simulink model "PM_block_control_FAST_syn_27_3"  (R2017a)
settings: Solver=ode4  StartTime=0.0  StopTime=100  FixedStep=0.0001  RelTol=1e-3
values from neighbouring files (symbols this model uses):
  Flux = 5.8264    [PM_1_5MW_syn_27.m]
  fs = 4000    [PM_1_5MW_syn_27.m]
  Id_set = 500    [PM_1_5MW_syn_27.m]
  Iq_set = 2200    [PM_1_5MW_syn_27.m]
  Ki = (Bandw/10*2*pi)*Kp    (= 0.0157079632679)    [PM_1_5MW_syn_27.m]
  Ki_Speed = Kp_Speed*2*pi*(BW/10)    (= 170820.076173)    [PM_1_5MW_syn_27.m]
  Kp = 1*.0005    (= 0.0005)    [PM_1_5MW_syn_27.m]
  Kp_Speed = 1.5*J/p*2*pi*BW    (= 5437.37190044)    [PM_1_5MW_syn_27.m]
  Ld = 0.001575    [PM_1_5MW_syn_27.m]
  Lq = 0.001575    [PM_1_5MW_syn_27.m]
  m = 1    [PM_1_5MW_syn_27.m]
  p = 26    [PM_1_5MW_syn_27.m]
  Rs = 0.000821    [PM_1_5MW_syn_27.m]
  Speed_set = w_m    (= 2.10172548525)    [PM_1_5MW_syn_27.m]
undefined symbols (not defined in the file or in its folder): Sollkurve_M_Optimum, Sollkurve_nGen_Optimum
libraries: powerlib x15, simulink x2
settings Model: Creator=Anjali  LastModifiedBy=sganzel
settings OptimizationCC: LifeSpan=inf
settings DebuggingCC: SFUnexpectedBacktrackingDiag=warning  SFNoUnconditionalDefaultTransitionDiag=warning  SFExecutionAtInitializationDiag=none
settings GRTTargetCC: TargetLangStandard=C89/C90 (ANSI)  GeneratePreprocessorConditionals=Disable all
settings ConfigComp: CovMetricSettings=dw  CovHtmlReporting=on  CovSaveCumulativeToWorkspaceVar=on  CovSaveSingleToWorkspaceVar=on  CovExternalEMLEnable=off

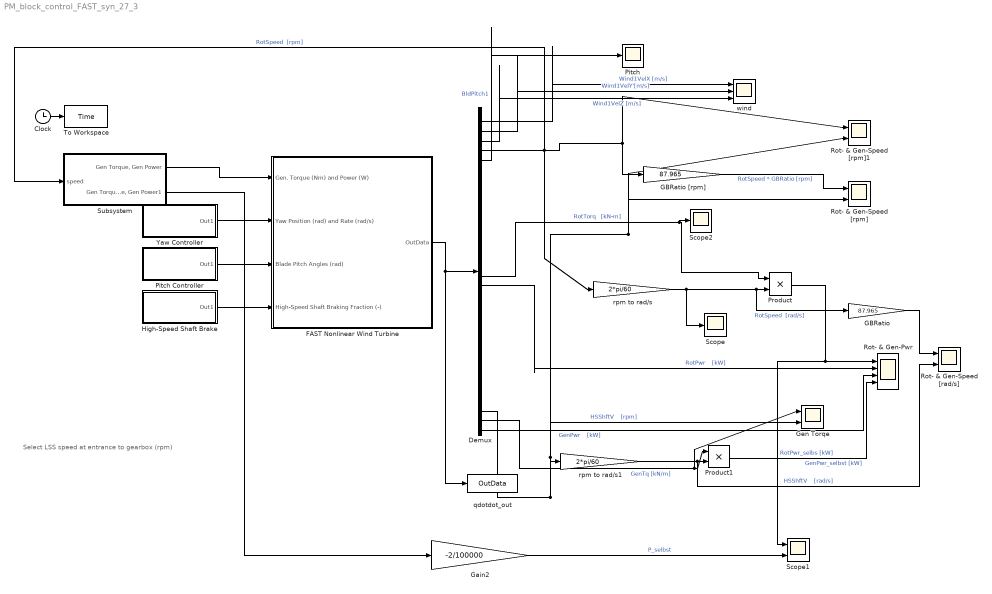
== system PM_block_control_FAST_syn_27_3 ==
  note: Select LSS speed at entrance to gearbox (rpm)
  Clock : Clock
  Demux : Demux  Outputs=34
  FAST Nonlinear Wind Turbine : Subsystem  mask(FAST Nonlinear Wind Turbine){}
      mask help: This block contains the FAST S-Function.
      mask init:
      | clear FAST_SFunc
  GBRatio : Gain  Gain=87.965
  GBRatio [rpm] : Gain  Gain=87.965
  Gain2 : Gain  Gain=-2/100000
  Gen Torqe : Scope  NumInputPorts=2
  High-Speed Shaft Brake : Subsystem
  Pitch : Scope
  Pitch Controller : Subsystem
  Product : Product
  Product1 : Product
  Rot- & Gen-Pwr : Scope  NumInputPorts=4
  Rot- & Gen-Speed [rad/s] : Scope  NumInputPorts=2
  Rot- & Gen-Speed [rpm] : Scope  NumInputPorts=2
  Rot- & Gen-Speed [rpm]1 : Scope  NumInputPorts=2
  Scope : Scope
  Scope1 : Scope  NumInputPorts=2
  Scope2 : Scope
  Subsystem : Subsystem
  To Workspace : ToWorkspace  VariableName=Time  SampleTime=-1
  Yaw Controller : Subsystem
  qdotdot_out : ToWorkspace  VariableName=OutData  SampleTime=-1
  rpm to rad/s : Gain  Gain=2*pi/60
  rpm to rad/s1 : Gain  Gain=2*pi/60
  wind : Scope  NumInputPorts=3
  wires:
  Clock/1 -> To Workspace/1
  Yaw Controller/1(Out1) -> FAST Nonlinear Wind Turbine/2(Yaw Position (rad) and Rate (rad/s))
  Pitch Controller/1(Out1) -> FAST Nonlinear Wind Turbine/3(Blade Pitch Angles (rad))
  FAST Nonlinear Wind Turbine/1(OutData) -> qdotdot_out/1, Demux/1
  High-Speed Shaft Brake/1(Out1) -> FAST Nonlinear Wind Turbine/4(High-Speed Shaft Braking Fraction (-))
  Demux/32 -> Gen Torqe/2, Rot- & Gen-Speed [rpm]1/2, Rot- & Gen-Speed [rpm]/2, rpm to rad/s1/1  "HSShftV    [rpm]"
  Demux/19 -> Rot- & Gen-Pwr/2  "RotPwr    [kW]"
  Demux/5 -> Rot- & Gen-Speed [rpm]1/1, GBRatio [rpm]/1, rpm to rad/s/1, Subsystem/1(speed)  "RotSpeed  [rpm]"
  Demux/18 -> Product/1, Scope2/1  "RotTorq   [kN-m]"
  Product/1 -> Scope1/1, Rot- & Gen-Pwr/1  "RotPwr_selbs [kW]"
  rpm to rad/s/1 -> Scope/1, GBRatio/1, Product/2  "RotSpeed  [rad/s]"
  Demux/34 -> Rot- & Gen-Pwr/3  "GenPwr    [kW]"
  Demux/33 -> Gen Torqe/1, Product1/1  "GenTq [kN/m]"
  rpm to rad/s1/1 -> Rot- & Gen-Speed [rad/s]/2, Product1/2  "HSShftV    [rad/s]"
  Product1/1 -> Rot- & Gen-Pwr/4  "GenPwr_selbst [kW]"
  GBRatio/1 -> Rot- & Gen-Speed [rad/s]/1
  GBRatio [rpm]/1 -> Rot- & Gen-Speed [rpm]/1  "RotSpeed * GBRatio [rpm]"
  Demux/2 -> wind/1  "Wind1VelX [m/s]"
  Demux/3 -> wind/2  "Wind1VelY [m/s]"
  Demux/4 -> wind/3  "Wind1VelZ [m/s]"
  Demux/6 -> Pitch/1  "BldPitch1"
  Subsystem/2("Gen Torque, Gen Power1") -> Gain2/1
  Gain2/1 -> Scope1/2  "P_selbst"
  Subsystem/1("Gen Torque, Gen Power") -> FAST Nonlinear Wind Turbine/1(Gen. Torque (Nm) and Power (W))

== system PM_block_control_FAST_syn_27_3/FAST Nonlinear Wind Turbine ==
  Gen. Torque (Nm) and Power (W) : Inport
  Yaw Position (rad) and Rate (rad/s) : Inport  Port=2
  Blade Pitch Angles (rad) : Inport  Port=3
  High-Speed Shaft Braking Fraction (-) : Inport  Port=4
  Mux1 : Mux
  S-Function : S-Function  FunctionName=FAST_SFunc  Parameters=FAST_InputFileName, TMax, 0  SFunctionDeploymentMode=off  EnableBusSupport=off
  Signal Specification1 : SignalSpecification  OutDataTypeStr=double  Dimensions=2
  Signal Specification2 : SignalSpecification  OutDataTypeStr=double  Dimensions=2
  OutData : Outport
  wires:
  Gen. Torque (Nm) and Power (W)/1 -> Signal Specification1/1
  S-Function/1 -> OutData/1
  Mux1/1 -> S-Function/1
  Blade Pitch Angles (rad)/1 -> Mux1/3
  Yaw Position (rad) and Rate (rad/s)/1 -> Signal Specification2/1
  Signal Specification1/1 -> Mux1/1
  Signal Specification2/1 -> Mux1/2
  High-Speed Shaft Braking Fraction (-)/1 -> Mux1/4

== system PM_block_control_FAST_syn_27_3/High-Speed Shaft Brake ==
  High-Speed Shaft Braking Fraction : Constant  Value=0
  Out1 : Outport
  wires:
  High-Speed Shaft Braking Fraction/1 -> Out1/1

== system PM_block_control_FAST_syn_27_3/Pitch Controller ==
  Blade Pitch Angles : Constant  Value=ones(1,3)'
  Pitch-winkel : Gain  Gain=0
  dergree2rad : Gain  Gain=2*pi/360
  Out1 : Outport
  wires:
  Blade Pitch Angles/1 -> Pitch-winkel/1
  Pitch-winkel/1 -> dergree2rad/1
  dergree2rad/1 -> Out1/1

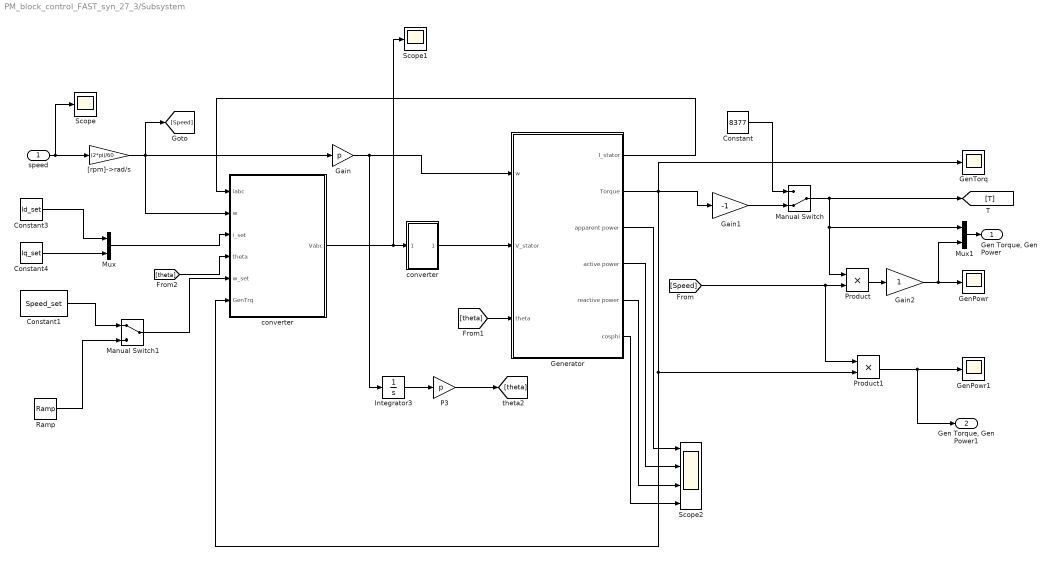
== system PM_block_control_FAST_syn_27_3/Subsystem ==
  speed : Inport
  Constant : Constant  Value=8377  VectorParams1D=off
  Constant1 : Constant  Value=Speed_set
  Constant3 : Constant  Value=Id_set
  Constant4 : Constant  Value=Iq_set
  Gain : Gain  Gain=p
  Gain1 : Gain  Gain=-1
  Gain2 : Gain
  GenPowr : Scope
  GenPowr1 : Scope
  GenTorq : Scope
  "Generator " : Subsystem
  Integrator3 : Integrator
  Manual Switch : ManualSwitch  CurrentSetting=0
  Manual Switch1 : ManualSwitch
  Mux : Mux  Inputs=2
  Mux1 : Mux  Inputs=2
  P3 : Gain  Gain=p
  Product : Product
  Product1 : Product
  Ramp : simulink/Sources/Ramp  slope=1/60*2*pi/10  start=40  X0=1.831548517042849
  Scope : Scope
  Scope1 : Scope
  Scope2 : Scope  NumInputPorts=4
  "[rpm]->rad/s" : Gain  Gain=(2*pi)/60
  converter : Subsystem
  "converter " : Subsystem
  "Gen Torque, Gen Power" : Outport
  "Gen Torque, Gen Power1" : Outport  Port=2
  wires:
  speed/1 -> Scope/1, "[rpm]->rad/s"/1
  "Generator "/1("I_stator ") -> "converter "/1(iabc)
  Constant3/1 -> Mux/1
  "Generator "/5(reactive power) -> Scope2/3
  [theta] -> "converter "/4(theta)
  Constant4/1 -> Mux/2
  "Generator "/6(cosphi) -> Scope2/4
  "Generator "/3(apparent power) -> Scope2/1
  "converter "/1(Vabc) -> Scope1/1, converter/1(iabc)
  "Generator "/4(active power) -> Scope2/2
  Constant1/1 -> Manual Switch1/1
  [theta] -> "Generator "/3("theta ")
  Mux/1 -> "converter "/3(i_set)
  Gain/1 -> Integrator3/1, "Generator "/1(w)
  "[rpm]->rad/s"/1 -> [Speed], Gain/1, "converter "/2(w)
  Integrator3/1 -> P3/1
  P3/1 -> [theta]
  [Speed] -> Product/2, Product1/1
  Product1/1 -> "Gen Torque, Gen Power1"/1, GenPowr1/1
  Mux1/1 -> "Gen Torque, Gen Power"/1
  Product/1 -> Gain2/1
  Constant/1 -> Manual Switch/1
  Gain2/1 -> GenPowr/1, Mux1/2
  "Generator "/2(Torque) -> Gain1/1, "converter "/6(GenTrq), Product1/2, GenTorq/1
  Manual Switch/1 -> [T], Mux1/1, Product/1
  Manual Switch1/1 -> "converter "/5(w_set)
  Ramp/1 -> Manual Switch1/2
  Gain1/1 -> Manual Switch/2
  converter/1(v_abc) -> "Generator "/2("V_stator ")

== system PM_block_control_FAST_syn_27_3/Yaw Controller ==
  Mux : Mux  Inputs=2
  Yaw Position : Constant  Value=0
  Yaw rate : Constant  Value=0
  Out1 : Outport
  wires:
  Mux/1 -> Out1/1
  Yaw Position/1 -> Mux/1
  Yaw rate/1 -> Mux/2

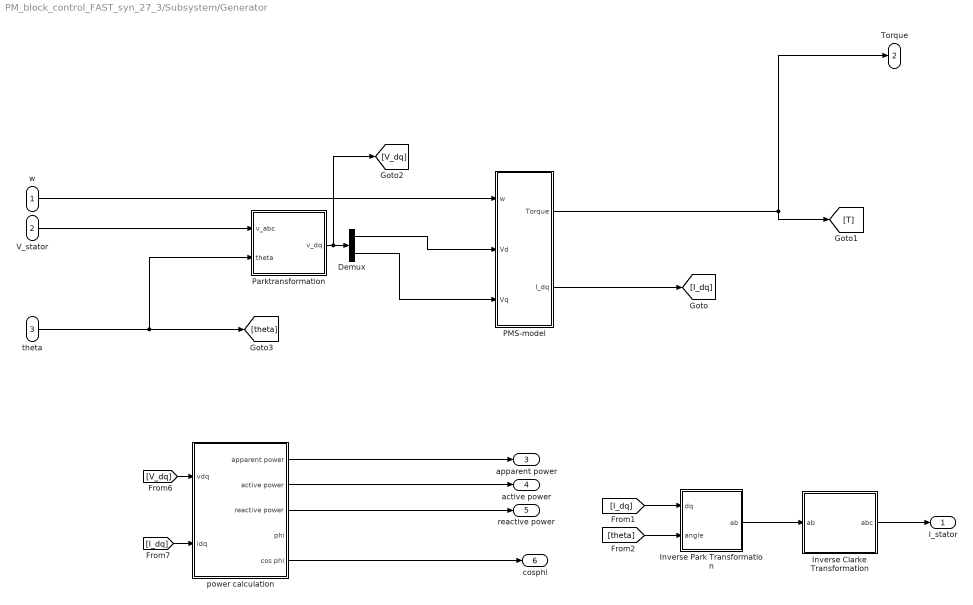
== system PM_block_control_FAST_syn_27_3/Subsystem/Generator  ==
  w : Inport
  "V_stator " : Inport  Port=2
  "theta " : Inport  Port=3
  Demux : Demux  Outputs=2
  Inverse Clarke Transformation : Subsystem
  Inverse Park Transformation : Subsystem
  PMS-model : Subsystem
  Parktransformation : Subsystem
  power calculation : Subsystem
  "I_stator " : Outport
  Torque : Outport  Port=2
  apparent power : Outport  Port=3
  active power : Outport  Port=4
  reactive power : Outport  Port=5
  cosphi : Outport  Port=6
  wires:
  PMS-model/2(I_dq) -> [I_dq]
  PMS-model/1(Torque) -> [T], Torque/1
  "V_stator "/1 -> Parktransformation/1(v_abc)
  "theta "/1 -> [theta], Parktransformation/2(theta)
  Parktransformation/1(v_dq) -> [V_dq], Demux/1
  Demux/1 -> PMS-model/2(Vd)
  Demux/2 -> PMS-model/3(Vq)
  w/1 -> PMS-model/1(w)
  Inverse Park Transformation/1(ab) -> Inverse Clarke Transformation/1(ab)
  [I_dq] -> Inverse Park Transformation/1(dq)
  Inverse Clarke Transformation/1(abc) -> "I_stator "/1
  [theta] -> Inverse Park Transformation/2(angle)
  [V_dq] -> power calculation/1(vdq)
  [I_dq] -> power calculation/2(idq)
  power calculation/3(reactive power) -> reactive power/1
  power calculation/2(active power) -> active power/1
  power calculation/1(apparent power) -> apparent power/1
  power calculation/5(cos phi) -> cosphi/1

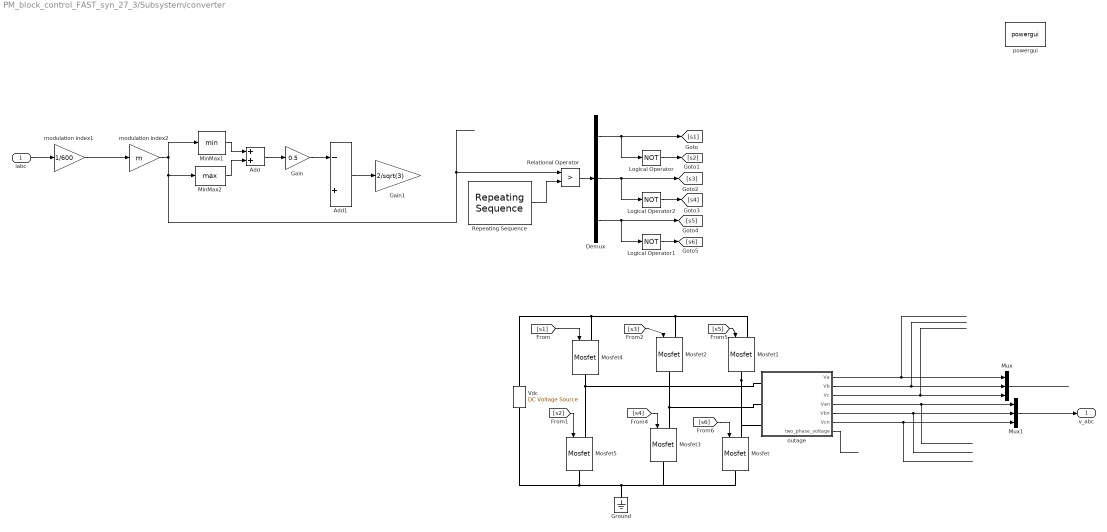
== system PM_block_control_FAST_syn_27_3/Subsystem/converter ==
  iabc : Inport
  Add : Sum
  Add1 : Sum  Inputs=-+
  Demux : Demux  Outputs=3
  Gain : Gain  Gain=0.5
  Gain1 : Gain  Gain=2/sqrt(3)
  Ground : powerlib/Elements/Ground  LConnTagsString=a
  Logical Operator : Logic  Operator=NOT  AllPortsSameDT=off  OutDataTypeStr=boolean
  Logical Operator1 : Logic  Operator=NOT  AllPortsSameDT=off  OutDataTypeStr=boolean
  Logical Operator2 : Logic  Operator=NOT  AllPortsSameDT=off  OutDataTypeStr=boolean
  MinMax1 : MinMax  SaturateOnIntegerOverflow=on  InputSameDT=on
  MinMax2 : MinMax  Function=max  SaturateOnIntegerOverflow=on  InputSameDT=on
  Mosfet{,1..5} (6 alike) : powerlib/Power Electronics/Mosfet  Ron=0.1  Lon=0  Rd=0.01  Vfd=0  IC=0  Rs=1e5  Cs=inf  Measurements=off
  Mux : Mux  Inputs=3
  Mux1 : Mux  Inputs=3
  Relational Operator : RelationalOperator  Operator=>  RndMeth=Nearest
  Repeating Sequence : simulink/Sources/Repeating Sequence  rep_seq_t=[0 0.25/fs 0.5/fs 0.75/fs 1/fs]  rep_seq_y=[1 0 -1 0 1]
  Vdc : powerlib/Electrical Sources/DC Voltage Source  Amplitude=1200  Measurements=None
  modulation index1 : Gain  Gain=1/600  SaturateOnIntegerOverflow=on  OutDataTypeStr=Inherit: Same as input  ParamDataTypeStr=Inherit: Same as input
  modulation index2 : Gain  Gain=m  SaturateOnIntegerOverflow=on  OutDataTypeStr=Inherit: Same as input  ParamDataTypeStr=Inherit: Same as input
  outage : Subsystem
  powergui : powerlib/powergui  Priority=1  SimulationMode=Continuous  SampleTime=50e-6  frequency=60  Iterations=50  frequencyindice=0  Pbase=100e6  ErrMax=1e-4  UnitsV=kV  UnitsW=MW  buscounter=0  FunctionMessages=off  echomessages=off  EnableUseOfTLC=off  CurrentSourceSwitches=on  DisableSnubberDevices=off  DisableRonSwitches=off  DisableVfSwitches=off  DisplayEquations=off  SolverType=Tustin/Backward Euler (TBE)  Interpol=off  ExternalGateDelay=off  methode=off  Ts=100  x0status=blocks  SPID=off  SwTol=0  HookPort=off  RestoreLinks=warning  ResistiveCurrentMeasurement=off  Frange=[0:2:500]  Ylog=off  Xlog=on  ShowGrid=off  save=off  variable=ZData  structure=Filtered_voltages  ZoomFFT=off  StartTime=0.02  cycles=1  DisplayStyle=1  fundamental=50  FreqAxis=off  MaxFrequency=1000  frequencyindicesteady=1  RmsSteady=1  display=off
  v_abc : Outport
  wires:
  Mux/1 -> ?
  Add1/1 -> Gain1/1
  Gain/1 -> Add1/1
  MinMax2/1 -> Add/2
  Add/1 -> Gain/1
  iabc/1 -> modulation index1/1
  MinMax1/1 -> Add/1
  Demux/2 -> [s3], Logical Operator2/1
  Demux/3 -> [s5], Logical Operator1/1
  Logical Operator1/1 -> [s6]
  Logical Operator/1 -> [s2]
  Logical Operator2/1 -> [s4]
  Demux/1 -> [s1], Logical Operator/1
  modulation index2/1 -> MinMax1/1, Relational Operator/1, MinMax2/1
  Relational Operator/1 -> Demux/1
  Repeating Sequence/1 -> Relational Operator/2
  outage/2(Vb) -> Mux/2
  [s3] -> Mosfet2/1
  outage/1(Va) -> Mux/1
  [s6] -> Mosfet/1
  [s2] -> Mosfet5/1
  [s5] -> Mosfet1/1
  [s4] -> Mosfet3/1
  [s1] -> Mosfet4/1
  outage/3(Vc) -> Mux/3
  outage/7(two_phase_voltage) -> ?
  modulation index1/1 -> modulation index2/1
  outage/6(Vcn) -> Mux1/3
  Mux1/1 -> v_abc/1
  outage/5(Vbn) -> Mux1/2
  outage/4(Van) -> Mux1/1
  connections:
  Mosfet5/RConn1 -- Vdc/LConn1 -- Ground/LConn1 -- Mosfet/RConn1 -- Mosfet3/RConn1
  Mosfet1/LConn1 -- Vdc/RConn1 -- Mosfet4/LConn1 -- Mosfet2/LConn1
  Mosfet5/LConn1 -- outage/LConn1 -- Mosfet4/RConn1
  Mosfet2/RConn1 -- Mosfet3/LConn1 -- outage/LConn2
  Mosfet1/RConn1 -- outage/LConn3 -- Mosfet/LConn1

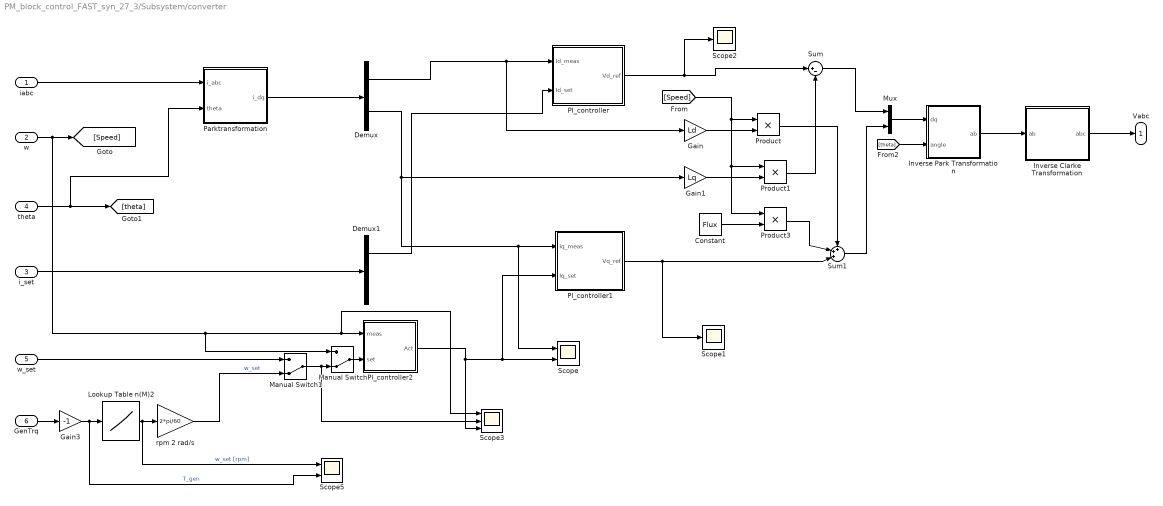
== system PM_block_control_FAST_syn_27_3/Subsystem/converter  ==
  iabc : Inport
  w : Inport  Port=2
  i_set : Inport  Port=3
  theta : Inport  Port=4
  w_set : Inport  Port=5
  GenTrq : Inport  Port=6
  Constant : Constant  Value=Flux
  Demux : Demux  Outputs=2
  Demux1 : Demux  Outputs=2
  Gain : Gain  Gain=Ld
  Gain1 : Gain  Gain=Lq
  Gain3 : Gain  Gain=-1
  Inverse Clarke Transformation : Subsystem
  Inverse Park Transformation : Subsystem
  Lookup Table n(M)2 : Lookup_n-D  NumberOfTableDimensions=1  BreakpointsForDimension1=Sollkurve_M_Optimum  Table=Sollkurve_nGen_Optimum  InternalRulePriority=Speed  RndMeth=Simplest  InputSameDT=on
  Manual Switch : ManualSwitch  CurrentSetting=0
  Manual Switch1 : ManualSwitch  CurrentSetting=0
  Mux : Mux  Inputs=2
  PI_controller : Subsystem
  PI_controller1 : Subsystem
  PI_controller2 : Subsystem
  Parktransformation : Subsystem
  Product : Product
  Product1 : Product
  Product3 : Product
  Scope : Scope  NumInputPorts=2
  Scope1 : Scope
  Scope2 : Scope
  Scope3 : Scope  NumInputPorts=3
  Scope5 : Scope  NumInputPorts=2
  Sum : Sum  Inputs=|+-
  Sum1 : Sum  Inputs=+++|
  rpm 2 rad/s : Gain  Gain=2*pi/60
  Vabc : Outport
  wires:
  iabc/1 -> Parktransformation/1(i_abc)
  Parktransformation/1(i_dq) -> Demux/1
  Demux/1 -> Gain/1, PI_controller/1(Id_meas)
  Demux/2 -> Gain1/1, Scope/1, PI_controller1/1(Iq_meas)
  i_set/1 -> Demux1/1
  Demux1/1 -> PI_controller/2(Id_set)
  Gain/1 -> Product/2
  Gain1/1 -> Product1/2
  [Speed] -> Product/1, Product3/1, Product1/1
  PI_controller/1(Vd_ref) -> Scope2/1, Sum/1
  Product1/1 -> Sum/2
  Product/1 -> Sum1/1
  Inverse Park Transformation/1(ab) -> Inverse Clarke Transformation/1(ab)
  Inverse Clarke Transformation/1(abc) -> Vabc/1
  Sum/1 -> Mux/1
  Sum1/1 -> Mux/2
  Mux/1 -> Inverse Park Transformation/1(dq)
  theta/1 -> Parktransformation/2(theta), [theta]
  [theta] -> Inverse Park Transformation/2(angle)
  PI_controller1/1(Vq_ref) -> Scope1/1, Sum1/3
  Constant/1 -> Product3/2
  Product3/1 -> Sum1/2
  w/1 -> Scope3/1, PI_controller2/1(meas), Manual Switch/1, [Speed]
  Manual Switch/1 -> PI_controller2/2(set)
  PI_controller2/1(Act) -> Scope/2, PI_controller1/2(Iq_set), Scope3/3
  Gain3/1 -> Scope5/2, Lookup Table n(M)2/1  "T_gen"
  rpm 2 rad/s/1 -> Manual Switch1/2  "w_set"
  w_set/1 -> Manual Switch1/1
  Manual Switch1/1 -> Scope3/2, Manual Switch/2
  Lookup Table n(M)2/1 -> Scope5/1, rpm 2 rad/s/1  "w_set [rpm]"
  GenTrq/1 -> Gain3/1

== system PM_block_control_FAST_syn_27_3/Subsystem/Generator /Inverse Clarke Transformation ==
  ab : Inport
  Demux : Demux  Outputs=2
  Gain1 : Gain  Gain=1/2
  Gain2 : Gain  Gain=sqrt(3)
  Gain4 : Gain  Gain=1/2
  Mux : Mux  Inputs=3
  Sum : Sum  Inputs=|-+
  Sum1 : Sum  Inputs=|--
  abc : Outport
  wires:
  Mux/1 -> abc/1
  ab/1 -> Demux/1
  Sum1/1 -> Gain1/1
  Sum/1 -> Gain4/1
  Gain2/1 -> Sum1/2, Sum/2
  Demux/1 -> Sum1/1, Sum/1, Mux/1
  Demux/2 -> Gain2/1
  Gain4/1 -> Mux/2
  Gain1/1 -> Mux/3

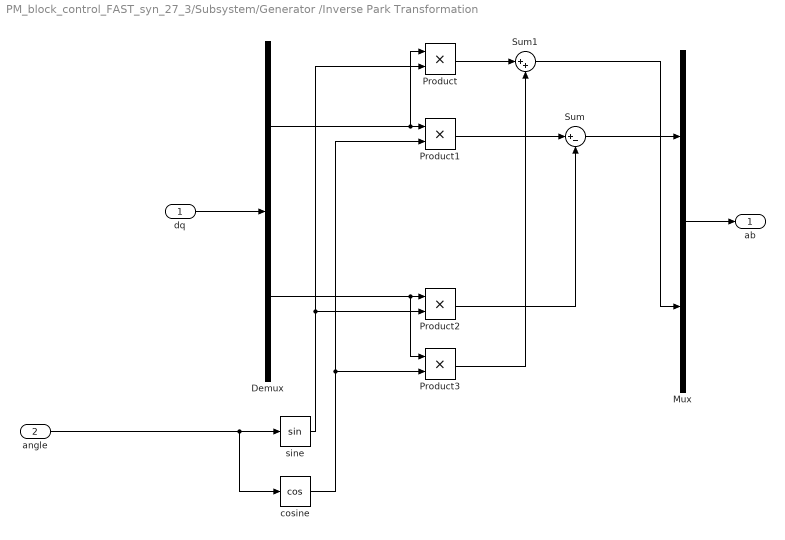
== system PM_block_control_FAST_syn_27_3/Subsystem/Generator /Inverse Park Transformation ==
  dq : Inport
  angle : Inport  Port=2
  Demux : Demux  Outputs=2
  Mux : Mux  Inputs=2
  Product{,1..3} (4 alike) : Product  RndMeth=Zero
  Sum : Sum  Inputs=|+-
  Sum1 : Sum  Inputs=|++
  cosine : Trigonometry  Operator=cos
  sine : Trigonometry
  ab : Outport
  wires:
  Sum1/1 -> Mux/2
  Sum/1 -> Mux/1
  Product2/1 -> Sum/2
  Product1/1 -> Sum/1
  Product3/1 -> Sum1/2
  Product/1 -> Sum1/1
  cosine/1 -> Product3/2, Product1/2
  sine/1 -> Product2/2, Product/2
  Demux/2 -> Product3/1, Product2/1
  Demux/1 -> Product1/1, Product/1
  Mux/1 -> ab/1
  dq/1 -> Demux/1
  angle/1 -> cosine/1, sine/1

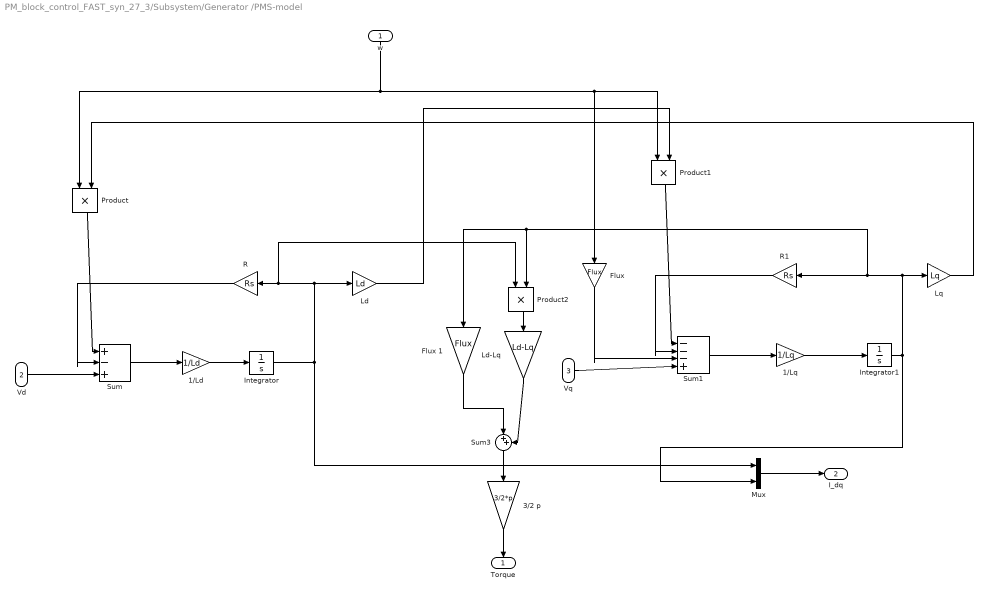
== system PM_block_control_FAST_syn_27_3/Subsystem/Generator /PMS-model ==
  w : Inport
  Vd : Inport  Port=2
  Vq : Inport  Port=3
  1/Ld : Gain  Gain=1/Ld
  1/Lq : Gain  Gain=1/Lq
  3/2 p : Gain  Gain=3/2*p
  "Flux " : Gain  Gain=Flux
  Flux 1 : Gain  Gain=Flux
  Integrator : Integrator
  Integrator1 : Integrator
  Ld : Gain  Gain=Ld
  Ld-Lq : Gain  Gain=Ld-Lq
  Lq : Gain  Gain=Lq
  Mux : Mux  Inputs=2
  Product : Product
  Product1 : Product
  Product2 : Product
  R : Gain  Gain=Rs
  R1 : Gain  Gain=Rs
  Sum : Sum  Inputs=|+-+
  Sum1 : Sum  Inputs=|---+
  Sum3 : Sum  Inputs=|++
  Torque : Outport
  I_dq : Outport  Port=2
  wires:
  R/1 -> Sum/2
  Product1/1 -> Sum1/1
  w/1 -> "Flux "/1, Product1/1, Product/1
  Vd/1 -> Sum/3
  3/2 p/1 -> Torque/1
  Mux/1 -> I_dq/1
  Product/1 -> Sum/1
  Sum3/1 -> 3/2 p/1
  R1/1 -> Sum1/2
  Sum/1 -> 1/Ld/1
  1/Ld/1 -> Integrator/1
  Integrator/1 -> Product2/1, R/1, Ld/1, Mux/1
  Sum1/1 -> 1/Lq/1
  1/Lq/1 -> Integrator1/1
  Integrator1/1 -> Product2/2, Flux 1/1, R1/1, Lq/1, Mux/2
  Ld/1 -> Product1/2
  Lq/1 -> Product/2
  Vq/1 -> Sum1/4
  "Flux "/1 -> Sum1/3
  Flux 1/1 -> Sum3/1
  Ld-Lq/1 -> Sum3/2
  Product2/1 -> Ld-Lq/1

== system PM_block_control_FAST_syn_27_3/Subsystem/Generator /Parktransformation ==
  v_abc : Inport
  theta : Inport  Port=2
  Scope1 : Scope
  Scope2 : Scope
  Scope3 : Scope
  Three-phase current : Subsystem
  abc to alpha-beta : Subsystem
  alpha-beta to dq : Subsystem
  f : Constant  Value=50
  f1 : Constant  Value=20
  v_dq : Outport
  wires:
  abc to alpha-beta/1("alpha-beta ") -> Scope1/1, alpha-beta to dq/2("alpha-beta ")
  alpha-beta to dq/1(Out1) -> v_dq/1, Scope2/1
  f1/1 -> Three-phase current/2(In2)
  v_abc/1 -> Scope3/1, abc to alpha-beta/1(abc)
  theta/1 -> alpha-beta to dq/1(theta)

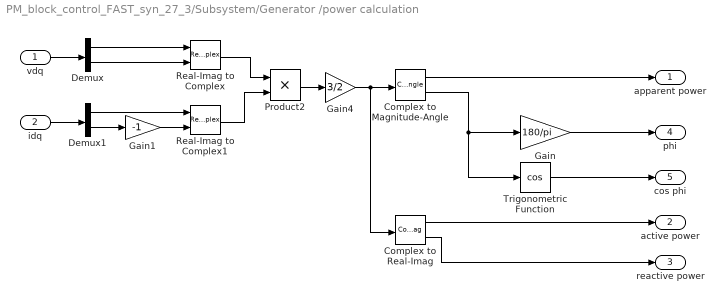
== system PM_block_control_FAST_syn_27_3/Subsystem/Generator /power calculation ==
  vdq : Inport
  idq : Inport  Port=2
  Complex to Magnitude-Angle : ComplexToMagnitudeAngle
  Complex to Real-Imag : ComplexToRealImag
  Demux : Demux  Outputs=2
  Demux1 : Demux  Outputs=2
  Gain : Gain  Gain=180/pi
  Gain1 : Gain  Gain=-1
  Gain4 : Gain  Gain=3/2
  Product2 : Product  RndMeth=Zero
  Real-Imag to Complex : RealImagToComplex
  Real-Imag to Complex1 : RealImagToComplex
  Trigonometric Function : Trigonometry  Operator=cos
  apparent power : Outport
  active power : Outport  Port=2
  reactive power : Outport  Port=3
  phi : Outport  Port=4
  cos phi : Outport  Port=5
  wires:
  Demux/1 -> Real-Imag to Complex/1
  Demux/2 -> Real-Imag to Complex/2
  Demux1/1 -> Real-Imag to Complex1/1
  Real-Imag to Complex/1 -> Product2/1
  Real-Imag to Complex1/1 -> Product2/2
  Product2/1 -> Gain4/1
  vdq/1 -> Demux/1
  idq/1 -> Demux1/1
  Complex to Magnitude-Angle/1 -> apparent power/1
  Complex to Magnitude-Angle/2 -> Trigonometric Function/1, Gain/1
  Gain/1 -> phi/1
  Demux1/2 -> Gain1/1
  Gain1/1 -> Real-Imag to Complex1/2
  Trigonometric Function/1 -> cos phi/1
  Complex to Real-Imag/1 -> active power/1
  Complex to Real-Imag/2 -> reactive power/1
  Gain4/1 -> Complex to Real-Imag/1, Complex to Magnitude-Angle/1

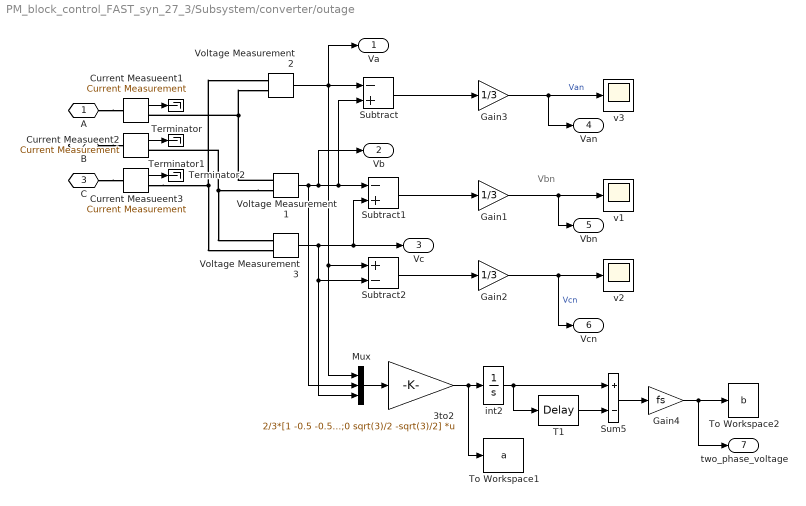
== system PM_block_control_FAST_syn_27_3/Subsystem/converter/outage ==
  note: Vbn
  3to2 : Gain  Gain=2/3*[1 -0.5 -0.5;0 sqrt(3)/2 -sqrt(3)/2]  Multiplication=Matrix(K*u)  SaturateOnIntegerOverflow=on  OutDataTypeStr=Inherit: Same as input  ParamDataTypeStr=Inherit: Same as input
  Current Measueent1 : powerlib/Measurements/Current Measurement  PhasorSimulation=off  OutputType=Complex  PSBequivalent=0
  Current Measueent2 : powerlib/Measurements/Current Measurement  PhasorSimulation=off  OutputType=Complex  PSBequivalent=0
  Current Measueent3 : powerlib/Measurements/Current Measurement  PhasorSimulation=off  OutputType=Complex  PSBequivalent=0
  Gain1 : Gain  Gain=1/3
  Gain2 : Gain  Gain=1/3
  Gain3 : Gain  Gain=1/3
  Gain4 : Gain  Gain=fs  SaturateOnIntegerOverflow=on  OutDataTypeStr=Inherit: Same as input  ParamDataTypeStr=Inherit: Same as input
  Mux : Mux  Inputs=3
  Subtract : Sum  Inputs=-+
  Subtract1 : Sum  Inputs=-+
  Subtract2 : Sum  Inputs=+-
  Sum5 : Sum  Inputs=+-  SaturateOnIntegerOverflow=on  InputSameDT=on  OutDataTypeStr=Inherit: Same as first input
  T1 : TransportDelay  DelayTime=1/fs  BufferSize=2048
  Terminator : Terminator
  Terminator1 : Terminator
  Terminator2 : Terminator
  To Workspace1 : ToWorkspace  VariableName=a  SampleTime=-1
      settings: Decimation=2
  To Workspace2 : ToWorkspace  VariableName=b  SampleTime=-1
      settings: Decimation=2
  Voltage Measurement1 : powerlib/Measurements/Voltage Measurement  PhasorSimulation=off  OutputType=Complex  PSBequivalent=0
  Voltage Measurement2 : powerlib/Measurements/Voltage Measurement  PhasorSimulation=off  OutputType=Complex  PSBequivalent=0
  Voltage Measurement3 : powerlib/Measurements/Voltage Measurement  PhasorSimulation=off  OutputType=Complex  PSBequivalent=0
  int2 : Integrator
  v1 : Scope
  v2 : Scope
  v3 : Scope
  A : PMIOPort  Port=1  Side=Left
  B : PMIOPort  Port=2  Side=Left
  C : PMIOPort  Port=3  Side=Left
  Va : Outport
  Vb : Outport  Port=2
  Vc : Outport  Port=3
  Van : Outport  Port=4
  Vbn : Outport  Port=5
  Vcn : Outport  Port=6
  two_phase_voltage : Outport  Port=7
  wires:
  Gain2/1 -> v2/1, Vcn/1  "Vcn"
  Subtract2/1 -> Gain2/1
  Gain1/1 -> v1/1, Vbn/1
  Subtract1/1 -> Gain1/1
  Voltage Measurement3/1 -> Subtract1/2, Vc/1, Subtract2/2, Mux/3
  Gain3/1 -> v3/1, Van/1  "Van"
  Subtract/1 -> Gain3/1
  Voltage Measurement1/1 -> Subtract/2, Subtract1/1, Vb/1, Mux/2
  Voltage Measurement2/1 -> Subtract/1, Va/1, Subtract2/1, Mux/1
  Current Measueent1/1 -> Terminator/1
  Current Measueent2/1 -> Terminator1/1
  Current Measueent3/1 -> Terminator2/1
  Mux/1 -> 3to2/1
  3to2/1 -> int2/1, To Workspace1/1
  T1/1 -> Sum5/2
  int2/1 -> Sum5/1, T1/1
  Sum5/1 -> Gain4/1
  Gain4/1 -> To Workspace2/1, two_phase_voltage/1
  connections:
  Voltage Measurement1/LConn1 -- Current Measueent1/RConn1 -- Voltage Measurement2/LConn2
  Voltage Measurement1/LConn2 -- Current Measueent2/RConn1 -- Voltage Measurement3/LConn1
  Current Measueent3/RConn1 -- Voltage Measurement2/LConn1 -- Voltage Measurement3/LConn2
  A/RConn1 -- Current Measueent1/LConn1
  B/RConn1 -- Current Measueent2/LConn1
  C/RConn1 -- Current Measueent3/LConn1

== system PM_block_control_FAST_syn_27_3/Subsystem/converter /Inverse Clarke Transformation ==
  ab : Inport
  Demux : Demux  Outputs=2
  Gain1 : Gain  Gain=1/2
  Gain2 : Gain  Gain=sqrt(3)
  Gain4 : Gain  Gain=1/2
  Mux : Mux  Inputs=3
  Sum : Sum  Inputs=|-+
  Sum1 : Sum  Inputs=|--
  abc : Outport
  wires:
  Mux/1 -> abc/1
  ab/1 -> Demux/1
  Sum1/1 -> Gain1/1
  Sum/1 -> Gain4/1
  Gain2/1 -> Sum1/2, Sum/2
  Demux/1 -> Sum1/1, Sum/1, Mux/1
  Demux/2 -> Gain2/1
  Gain4/1 -> Mux/2
  Gain1/1 -> Mux/3

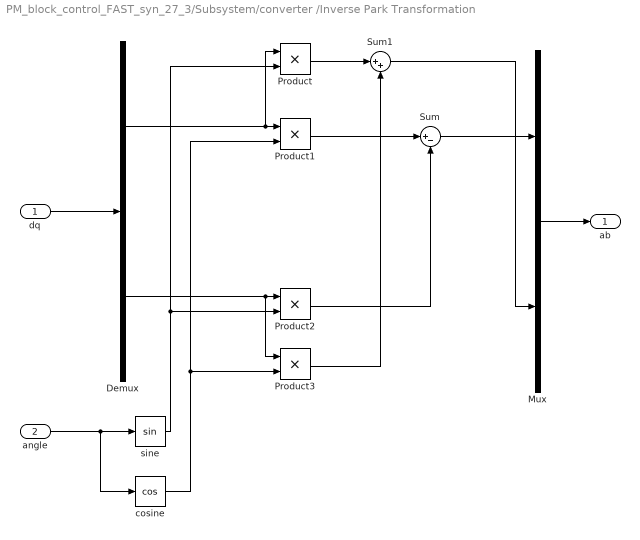
== system PM_block_control_FAST_syn_27_3/Subsystem/converter /Inverse Park Transformation ==
  dq : Inport
  angle : Inport  Port=2
  Demux : Demux  Outputs=2
  Mux : Mux  Inputs=2
  Product{,1..3} (4 alike) : Product  RndMeth=Zero
  Sum : Sum  Inputs=|+-
  Sum1 : Sum  Inputs=|++
  cosine : Trigonometry  Operator=cos
  sine : Trigonometry
  ab : Outport
  wires:
  Sum1/1 -> Mux/2
  Sum/1 -> Mux/1
  Product2/1 -> Sum/2
  Product1/1 -> Sum/1
  Product3/1 -> Sum1/2
  Product/1 -> Sum1/1
  angle/1 -> cosine/1, sine/1
  cosine/1 -> Product3/2, Product1/2
  sine/1 -> Product2/2, Product/2
  Demux/2 -> Product3/1, Product2/1
  Demux/1 -> Product1/1, Product/1
  Mux/1 -> ab/1
  dq/1 -> Demux/1

== system PM_block_control_FAST_syn_27_3/Subsystem/converter /PI_controller ==
  Id_meas : Inport
  Id_set : Inport  Port=2
  Gain : Gain  Gain=Kp
  Gain1 : Gain  Gain=Ki
  Integrator : Integrator
  Sum : Sum  Inputs=|++
  Sum1 : Sum  Inputs=|-+
  "id " : Scope  NumInputPorts=2
  Vd_ref : Outport
  wires:
  Gain/1 -> Sum/1
  Integrator/1 -> Sum/2
  Sum1/1 -> Gain1/1, Gain/1
  Id_meas/1 -> "id "/1, Sum1/1
  Id_set/1 -> "id "/2, Sum1/2
  Sum/1 -> Vd_ref/1
  Gain1/1 -> Integrator/1

== system PM_block_control_FAST_syn_27_3/Subsystem/converter /PI_controller1 ==
  Iq_meas : Inport
  Iq_set : Inport  Port=2
  Gain : Gain  Gain=Kp
  Gain1 : Gain  Gain=Ki
  Integrator : Integrator
  Sum : Sum  Inputs=|++
  Sum1 : Sum  Inputs=|-+
  iq : Scope  NumInputPorts=2
  Vq_ref : Outport
  wires:
  Gain1/1 -> Integrator/1
  Sum/1 -> Vq_ref/1
  Iq_set/1 -> iq/1, Sum1/2
  Sum1/1 -> Gain/1, Gain1/1
  Integrator/1 -> Sum/2
  Gain/1 -> Sum/1
  Iq_meas/1 -> iq/2, Sum1/1

== system PM_block_control_FAST_syn_27_3/Subsystem/converter /PI_controller2 ==
  meas : Inport
  set : Inport  Port=2
  Gain : Gain  Gain=Kp_Speed
  Gain1 : Gain  Gain=Ki_Speed
  Integrator : Integrator
  Sum : Sum  Inputs=|++
  Sum1 : Sum  Inputs=|-+
  "speed " : Scope  NumInputPorts=2
  Act : Outport
  wires:
  Gain1/1 -> Integrator/1
  Sum/1 -> Act/1
  Sum1/1 -> Gain1/1, Gain/1
  Integrator/1 -> Sum/2
  Gain/1 -> Sum/1
  set/1 -> "speed "/1, Sum1/2
  meas/1 -> "speed "/2, Sum1/1

== system PM_block_control_FAST_syn_27_3/Subsystem/converter /Parktransformation ==
  i_abc : Inport
  theta : Inport  Port=2
  3phase to ab : Subsystem
  alpha-beta to dq : Subsystem
  i_dq : Outport
  wires:
  3phase to ab/1(Out1) -> alpha-beta to dq/2("alpha-beta ")
  alpha-beta to dq/1(Out1) -> i_dq/1
  i_abc/1 -> 3phase to ab/1(In1)
  theta/1 -> alpha-beta to dq/1(theta)

== system PM_block_control_FAST_syn_27_3/Subsystem/Generator /Parktransformation/Three-phase current ==
  In1 : Inport
  In2 : Inport  Port=2
  Constant3 : Constant  Value=2*pi/3
  Constant4 : Constant  Value=-2*pi/3
  Gain : Gain  Gain=2*pi
  Integrator : Integrator
  Mux : Mux  Inputs=3
  Product : Product
  Sum : Sum  Inputs=|++
  Sum1 : Sum  Inputs=|++
  Trigonometric Function : Trigonometry  Operator=cos
  "abc " : Outport
  wires:
  Constant4/1 -> Sum1/2
  Trigonometric Function/1 -> Product/1
  Gain/1 -> Integrator/1
  In1/1 -> Gain/1
  In2/1 -> Product/2
  Sum/1 -> Mux/2
  Constant3/1 -> Sum/2
  Sum1/1 -> Mux/3
  Mux/1 -> Trigonometric Function/1
  Integrator/1 -> Sum/1, Sum1/1, Mux/1
  Product/1 -> "abc "/1

== system PM_block_control_FAST_syn_27_3/Subsystem/Generator /Parktransformation/abc to alpha-beta ==
  abc : Inport
  Demux : Demux  Outputs=3
  Gain : Gain  Gain=1/sqrt(3)
  Mux : Mux  Inputs=2
  Sum : Sum  Inputs=|+-
  "alpha-beta " : Outport
  wires:
  abc/1 -> Demux/1
  Sum/1 -> Gain/1
  Demux/2 -> Sum/1
  Demux/3 -> Sum/2
  Gain/1 -> Mux/2
  Demux/1 -> Mux/1
  Mux/1 -> "alpha-beta "/1

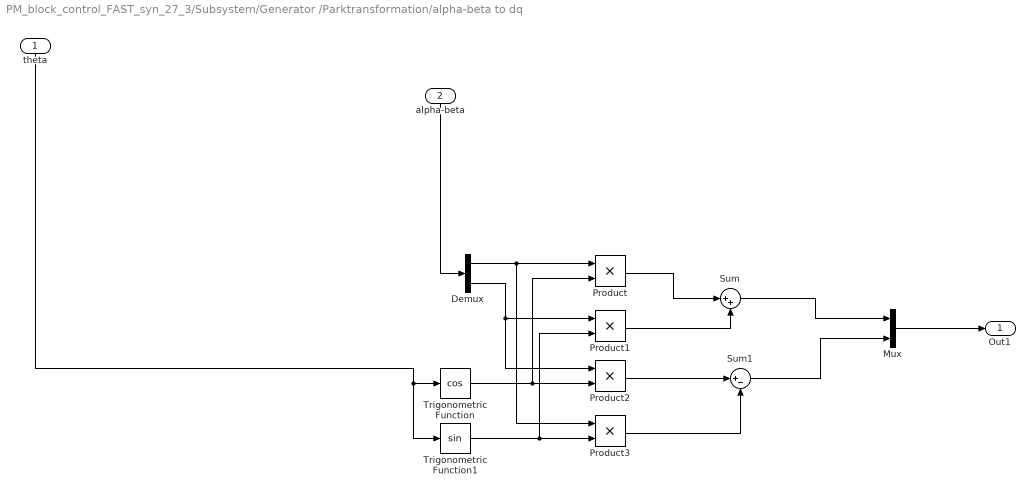
== system PM_block_control_FAST_syn_27_3/Subsystem/Generator /Parktransformation/alpha-beta to dq ==
  theta : Inport
  "alpha-beta " : Inport  Port=2
  Demux : Demux  Outputs=2
  Mux : Mux  Inputs=2
  Product{,1..3} (4 alike) : Product
  Sum : Sum  Inputs=|++
  Sum1 : Sum  Inputs=|+-
  Trigonometric Function : Trigonometry  Operator=cos
  Trigonometric Function1 : Trigonometry
  Out1 : Outport
  wires:
  Trigonometric Function1/1 -> Product3/2, Product1/2
  Product/1 -> Sum/1
  Product3/1 -> Sum1/2
  Product2/1 -> Sum1/1
  Sum/1 -> Mux/1
  Demux/1 -> Product3/1, Product/1
  Trigonometric Function/1 -> Product2/2, Product/2
  Demux/2 -> Product2/1, Product1/1
  Sum1/1 -> Mux/2
  Product1/1 -> Sum/2
  Mux/1 -> Out1/1
  "alpha-beta "/1 -> Demux/1
  theta/1 -> Trigonometric Function1/1, Trigonometric Function/1

== system PM_block_control_FAST_syn_27_3/Subsystem/converter /Parktransformation/3phase to ab ==
  In1 : Inport
  Demux : Demux  Outputs=3
  Gain3 : Gain  Gain=1/sqrt(3)
  Mux : Mux  Inputs=2
  Scope : Scope
  Sum1 : Sum  Inputs=|+-
  Out1 : Outport
  wires:
  Mux/1 -> Scope/1, Out1/1
  Demux/2 -> Sum1/1
  Demux/3 -> Sum1/2
  Sum1/1 -> Gain3/1
  In1/1 -> Demux/1
  Demux/1 -> Mux/1
  Gain3/1 -> Mux/2

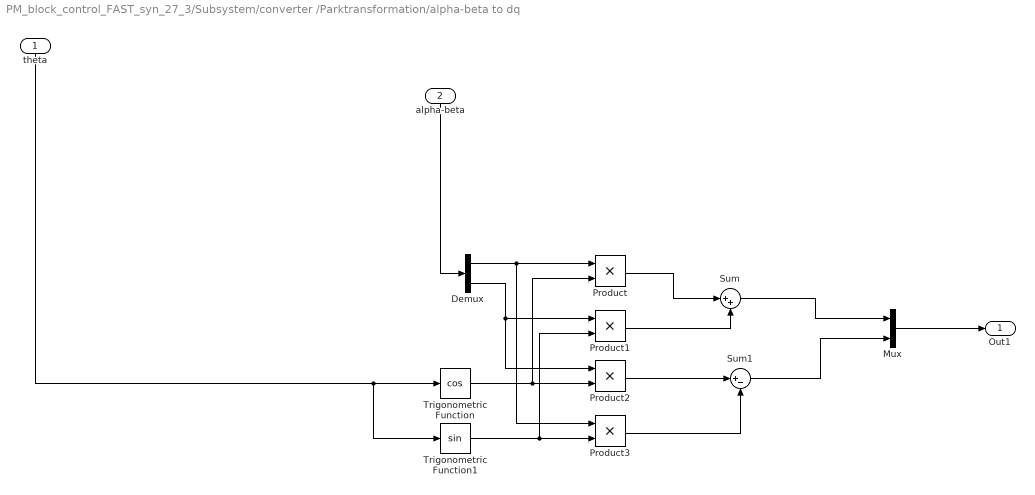
== system PM_block_control_FAST_syn_27_3/Subsystem/converter /Parktransformation/alpha-beta to dq ==
  theta : Inport
  "alpha-beta " : Inport  Port=2
  Demux : Demux  Outputs=2
  Mux : Mux  Inputs=2
  Product{,1..3} (4 alike) : Product
  Sum : Sum  Inputs=|++
  Sum1 : Sum  Inputs=|+-
  Trigonometric Function : Trigonometry  Operator=cos
  Trigonometric Function1 : Trigonometry
  Out1 : Outport
  wires:
  Trigonometric Function1/1 -> Product3/2, Product1/2
  Product/1 -> Sum/1
  Product3/1 -> Sum1/2
  Product2/1 -> Sum1/1
  Sum/1 -> Mux/1
  Demux/1 -> Product3/1, Product/1
  Trigonometric Function/1 -> Product2/2, Product/2
  Demux/2 -> Product2/1, Product1/1
  Sum1/1 -> Mux/2
  Product1/1 -> Sum/2
  Mux/1 -> Out1/1
  "alpha-beta "/1 -> Demux/1
  theta/1 -> Trigonometric Function1/1, Trigonometric Function/1
